simulink model "Cognata_Amp_Tobi_Split_Excel1"  (R2020a)
settings: Solver=VariableStepAuto  StartTime=0.0  StopTime=inf  RelTol=1e-3
model workspace (MAT data in the model file):
  WinSize = Simulink.Parameter
  WinSize.Value = 16
  WinSize.DataType = 'double'
  WinSize.Dimensions = [1 1]
  fc_bandpass = Simulink.Parameter
  fc_bandpass.Value = [0.05 0.26]
  fc_bandpass.DataType = 'double'
  fc_bandpass.Dimensions = [1 2]
undefined symbols (not defined in the file or in its folder): A1, A138674, A91496, C1, currentCFG_Cognata_Amp_Tobi_split_UB, I1, J138674, P91496, UB, W1, W91496
libraries: gtecHighspeedLib x1, gUSBamplib x1
settings Model: Creator=LAB-OREN3  LastModifiedBy=LAB-OREN3

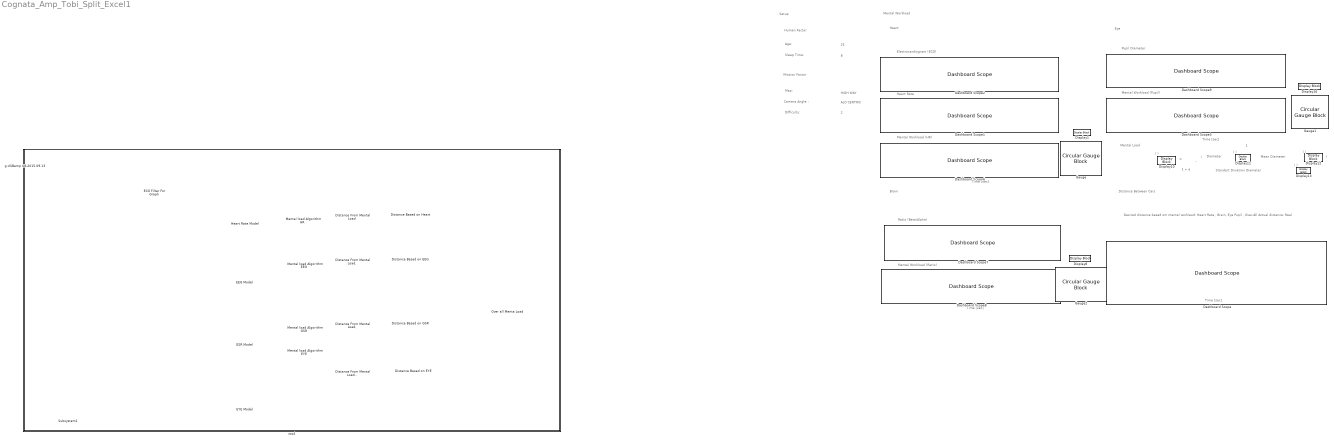
== system Cognata_Amp_Tobi_Split_Excel1 ==
  note: Mental Load
  note: Difficulty:
  note: Brain
  note: ( )
  note: ( )
  note: 1 + e
  note: . Setup
  note: Map:
  note: Diameter
  note: )
  note: Heart Rate
  note: Heart
  note: -
  note: ALO CENTRIC
  note: Time [sec]
  note: . Distance Between Cars
  note: Desired distance based om mental worklaod:
      | Heart Rate , Brain, Eye Pupil , Over-All
      |
      | Actual distance: Real
  note: HIGH WAY
  note: Sleep Time:
  note: 2
  note: Time [sec]
  note: Human Factor
  note: 1
  note: Electrocardiogram (ECG)
  note: Standart Diviation Diameter
  note: Mental Workload (HR)
  note: Ratio (Beta/Alpha)
  note: Time [sec]
  note: 25
  note: (
  note: 8
  note: Camera Angle: :
  note: Eye
  note: Mental Workload (Ratio)
  note: ( )
  note: =
  note: Pupil Diameter
  note: Mental Workload (Pupil)
  note: Time [sec]
  note: ( )
  note: Mission Factor
  note: Mean Diameter
  note: Mental Workload
  note: Age:
  Dashboard Scope : DashboardScope  ShowInitialText=off  TimeSpan=10  Ymin=-1  Ymax=20  LegendPosition=Hide  ScaleAtStop=off
  Dashboard Scope1 : DashboardScope  TimeSpan=10  Ymin=0  Ymax=100  LegendPosition=Hide  ScaleAtStop=off
  Dashboard Scope2 : DashboardScope  TimeSpan=10  Ymin=-3000  Ymax=1000  LegendPosition=Hide  ScaleAtStop=off
  Dashboard Scope3 : DashboardScope  TimeSpan=10  Ymin=0  Ymax=1  LegendPosition=Hide  ScaleAtStop=off
  Dashboard Scope6 : DashboardScope  TimeSpan=10  Ymin=0  Ymax=1  LegendPosition=Hide  ScaleAtStop=off
  Dashboard Scope7 : DashboardScope  TimeSpan=10  Ymin=0  Ymax=0.5  LegendPosition=Hide  ScaleAtStop=off
  Dashboard Scope8 : DashboardScope  TimeSpan=10  Ymin=0  Ymax=1  LegendPosition=Hide  ScaleAtStop=off
  Dashboard Scope9 : DashboardScope  TimeSpan=10  Ymin=0  Ymax=5  LegendPosition=Hide  ScaleAtStop=off
  Display{1,8,10..11,13,16} (6 alike) : DisplayBlock  LabelPosition=Hide  Format=bank  Transparency=1
  Display12 : DisplayBlock  LabelPosition=Hide  Format=bank  Transparency=1  Layout=Fill available space
  Distance Based on EEG : Display
  Distance Based on EYE : Display
  Distance Based on GSR : Display
  Distance Based on Heart : Display
  Distance From Mental Load : MATLAB Function  TreatAsAtomicUnit=on
  Distance From Mental Load, : MATLAB Function  TreatAsAtomicUnit=on
  Distance From Mental Load. : MATLAB Function  TreatAsAtomicUnit=on
  Distance From Mental Load.. : MATLAB Function  TreatAsAtomicUnit=on
  ECG Filter For Graph : Subsystem
  EEG Model : Subsystem  ReferencedSubsystem=EEG_Ratio_Model
  EYE Model : Subsystem  ReferencedSubsystem=Pupil_Diameter_Model
  GSR Model : Subsystem
  Gauge : CircularGaugeBlock  LabelPosition=Hide  ScaleMax=1  TickInterval=0.2
  Gauge1 : CircularGaugeBlock  LabelPosition=Hide  ScaleMax=1  TickInterval=0.2
  Gauge2 : CircularGaugeBlock  LabelPosition=Hide  ScaleMax=1  TickInterval=0.2
  Heart Rate Model : Subsystem  ReferencedSubsystem=Heart_Rate_Model
  Mental load Algorithm EEG : MATLAB Function  TreatAsAtomicUnit=on
  Mental load Algorithm EYE : MATLAB Function  TreatAsAtomicUnit=on
  Mental load Algorithm GSR : MATLAB Function  TreatAsAtomicUnit=on
  Mental load Algorithm HR : MATLAB Function  TreatAsAtomicUnit=on
  Over all Menta Load : Subsystem
  Subsystem1 : Subsystem
  g.USBamp UB-2015.09.13 : gUSBamplib/g.USBamp  cfg=currentCFG_Cognata_Amp_Tobi_split_UB-2015.09.13.cfg  snr=UB-2015.09.13
      settings: SourceProductName=g.USBamp
  zzz4 : Subsystem  TreatAsAtomicUnit=on
      settings: OpenFcn=% no-op
      mask Display: disp('')
  wires:
  Mental load Algorithm EEG/1(y) -> Distance From Mental Load./1(u), Over all Menta Load/2(Ratio)
  Distance From Mental Load/1(y) -> Distance Based on Heart/1
  Distance From Mental Load../1(y) -> Distance Based on EYE/1
  Mental load Algorithm HR/1(y) -> Distance From Mental Load/1(u), Over all Menta Load/1(HR)
  Distance From Mental Load./1(y) -> Distance Based on EEG/1
  Mental load Algorithm EYE/1(y) -> Distance From Mental Load../1(u), Over all Menta Load/4(eye)
  EEG Model/1 -> Mental load Algorithm EEG/1(u)
  EYE Model/1 -> Mental load Algorithm EYE/1(u)
  Heart Rate Model/2 -> Mental load Algorithm HR/1(u)
  Mental load Algorithm GSR/1(y) -> Distance From Mental Load,/1(u), Over all Menta Load/3(GSR)
  Distance From Mental Load,/1(y) -> Distance Based on GSR/1
  GSR Model/1(GSR) -> Mental load Algorithm GSR/1(u)
  Over all Menta Load/1(Over All Mental Load) -> ?
  EYE Model/2 -> ?
  EYE Model/3 -> ?
  Subsystem1/1("ECG, Without Filter") -> ECG Filter For Graph/1(In1), Heart Rate Model/1
  Subsystem1/2(EEG1) -> EEG Model/1
  Subsystem1/3(EEG2) -> EEG Model/2
  Subsystem1/4(EEG3) -> EEG Model/3
  Subsystem1/5(EEG4) -> EEG Model/4
  Subsystem1/6(EGG5) -> EEG Model/5
  Subsystem1/7(EEG 6) -> EEG Model/6
  Subsystem1/8(EEG 7) -> EEG Model/7
  Subsystem1/9(EEG8) -> EEG Model/8
  Subsystem1/10(EEG 9) -> EEG Model/9
  Subsystem1/11(EEG 19) -> EEG Model/10
  Subsystem1/12(EEG 11) -> EEG Model/11
  Subsystem1/14(GSR) -> GSR Model/1(In1)
  Subsystem1/15(Right Pupil Diameter) -> EYE Model/1
  Subsystem1/16(Left Pupil Diameter) -> EYE Model/2
  ECG Filter For Graph/1(EEG) -> ?
  Subsystem1/17(Distance From Simulator) -> ?
  Subsystem1/13(EEG 12) -> EEG Model/12

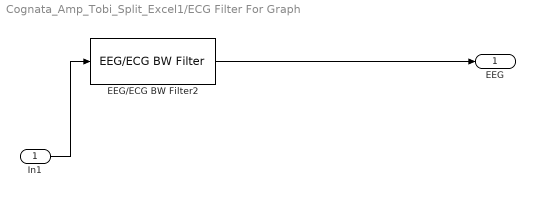
== system Cognata_Amp_Tobi_Split_Excel1/ECG Filter For Graph ==
  In1 : Inport
  EEG/ECG BW Filter2 : gtecHighspeedLib/EEG//ECG BW Filter  Order=6  LowerFreq=0.1  UpperFreq=30  SampFreq=512
      settings: SourceProductName=g.HIsys Library
  EEG : Outport
  wires:
  EEG/ECG BW Filter2/1 -> EEG/1
  In1/1 -> EEG/ECG BW Filter2/1

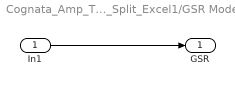
== system Cognata_Amp_Tobi_Split_Excel1/GSR Model ==
  In1 : Inport
  GSR : Outport
  wires:
  In1/1 -> GSR/1

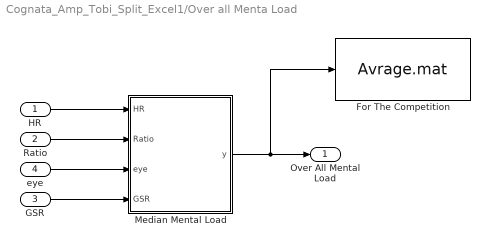
== system Cognata_Amp_Tobi_Split_Excel1/Over all Menta Load ==
  HR : Inport
  Ratio : Inport  Port=2
  GSR : Inport  Port=3
  eye : Inport  Port=4
  For The Competition : ToFile  Filename=Avrage.mat  MatrixName=Avrage
  Median Mental Load : MATLAB Function  TreatAsAtomicUnit=on
  Over All Mental Load : Outport
  wires:
  GSR/1 -> Median Mental Load/4(GSR)
  Median Mental Load/1(y) -> For The Competition/1, Over All Mental Load/1
  Ratio/1 -> Median Mental Load/2(Ratio)
  eye/1 -> Median Mental Load/3(eye)
  HR/1 -> Median Mental Load/1(HR)

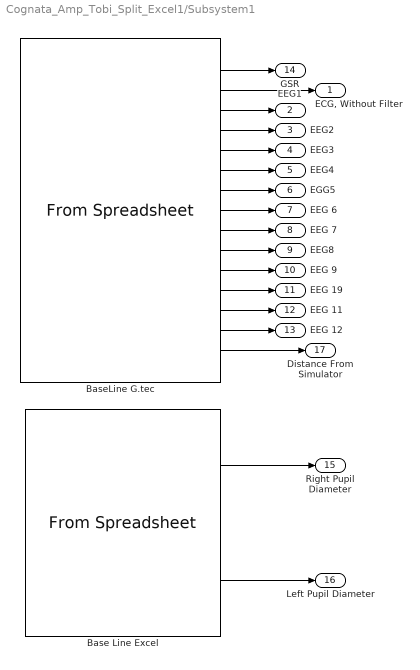
== system Cognata_Amp_Tobi_Split_Excel1/Subsystem1 ==
  Base Line Excel : FromSpreadsheet  FileName=C:\Users\LAB-OREN3\Downloads\1\Tobii Data of A2_535986_COMBINED_CUBE_DELAY_50_TTC_15 at (15;28;36).xlsx  SheetName=גיליון1  Range=A1:A138674,I1:J138674  SampleTime=0.001953125
  BaseLine G.tec : FromSpreadsheet  FileName=C:\Users\LAB-OREN3\Downloads\1\g.techAmp Data of A2_535986_COMBINED_CUBE_DELAY_50_TTC_15 at (15;28;36).xlsx  SheetName=גיליון1  Range=A1:A91496,C1:P91496,W1:W91496  SampleTime=0.001953125
  "ECG, Without Filter" : Outport
  EEG1 : Outport  Port=2
  EEG2 : Outport  Port=3
  EEG3 : Outport  Port=4
  EEG4 : Outport  Port=5
  EGG5 : Outport  Port=6
  EEG 6 : Outport  Port=7
  EEG 7 : Outport  Port=8
  EEG8 : Outport  Port=9
  EEG 9 : Outport  Port=10
  EEG 19 : Outport  Port=11
  EEG 11 : Outport  Port=12
  EEG 12 : Outport  Port=13
  GSR : Outport  Port=14
  Right Pupil Diameter : Outport  Port=15
  Left Pupil Diameter : Outport  Port=16
  Distance From Simulator : Outport  Port=17
  wires:
  BaseLine G.tec/5 -> EEG3/1
  BaseLine G.tec/13 -> EEG 11/1
  BaseLine G.tec/10 -> EEG8/1
  BaseLine G.tec/11 -> EEG 9/1
  BaseLine G.tec/14 -> EEG 12/1
  Base Line Excel/1 -> Right Pupil Diameter/1
  Base Line Excel/2 -> Left Pupil Diameter/1
  BaseLine G.tec/12 -> EEG 19/1
  BaseLine G.tec/8 -> EEG 6/1
  BaseLine G.tec/4 -> EEG2/1
  BaseLine G.tec/9 -> EEG 7/1
  BaseLine G.tec/6 -> EEG4/1
  BaseLine G.tec/1 -> GSR/1
  BaseLine G.tec/7 -> EGG5/1
  BaseLine G.tec/2 -> "ECG, Without Filter"/1
  BaseLine G.tec/3 -> EEG1/1
  BaseLine G.tec/15 -> Distance From Simulator/1

== system Cognata_Amp_Tobi_Split_Excel1/zzz4 ==

== matlab function Cognata_Amp_Tobi_Split_Excel1/Distance From Mental Load ==
  data: u input; y output
function y = fcn(u)
%#codegen

y = (u*10)+10;

== matlab function Cognata_Amp_Tobi_Split_Excel1/Mental load Algorithm HR ==
  data: u input; y output
function y = fcn(u)

y= probability_of_mental_load_HR(u);

end

== matlab function Cognata_Amp_Tobi_Split_Excel1/Over all Menta Load/Median Mental Load ==
  data: HR input; y output; Ratio input; eye input; GSR input
function y = fcn(HR, Ratio, eye, GSR)


    vac = [HR Ratio,eye,GSR];
    y = median(vac);

end

== matlab function Cognata_Amp_Tobi_Split_Excel1/Mental load Algorithm EEG ==
  data: u input; y output
function y = fcn(u)

y= probability_of_metal_load_EEG(u);

end

== matlab function Cognata_Amp_Tobi_Split_Excel1/Distance From Mental Load. ==
  data: u input; y output
function y = fcn(u)
%#codegen

y = (u*10)+10;

== matlab function Cognata_Amp_Tobi_Split_Excel1/Mental load Algorithm EYE ==
  data: u input; y output
function y = fcn( u)

y= probability_of_metal_load_EYE(u);

end

== matlab function Cognata_Amp_Tobi_Split_Excel1/Distance From Mental Load.. ==
  data: u input; y output
function y = fcn(u)
%#codegen

y = (u*10)+10;

== matlab function Cognata_Amp_Tobi_Split_Excel1/Mental load Algorithm GSR ==
  data: u input; y output
function y = fcn(u)

y= probability_of_metal_load_GSR(u);

end

== matlab function Cognata_Amp_Tobi_Split_Excel1/Distance From Mental Load, ==
  data: u input; y output
function y = fcn(u)
%#codegen

y = (u*10)+10;
